simulink model "reaction_pendulum_OBSERVERCOMP"  (R2021b)
settings: Solver=FixedStepDiscrete  StartTime=0.0  StopTime=inf  FixedStep=h  RelTol=1e-3  EnableMultiTasking=on
PreLoadFcn:
  | warning('off','MATLAB:dispatcher:InexactMatch');
InitFcn:
  | hwinit
values from neighbouring files (symbols this model uses):
  A = [0.989609173212  0  0; 0  1  0.01; -0.000301949872013  -0.0950246262215  0.997224421049]    [MATRICES.mat]    (also in SS_11_5.mat = [0.9904  0  0; 0  1  0.01; -9e-05  -0.033262024  0.99812133]; WEAREGOINGHOMEMATRICES.mat = [0.989609173212  0  0; 0  1  0.01; 0.000423899858033  -0.095; current_SS.mat = [0.989609173212  0  0; 0  1  0.01; -9.34612180115e-05  -0.02; dynamicUpdateModel.m = [1.000494318995348 0.010001647563961 2.391143629140888e-07)
  Aeq = [Aeq; Ax0]    [Manual_MPC_Companion.m]    (also in Manual_MPC_Companion_THURSDAY.m = zeros(n * Np, n_total))
  B = [4.20519003073 0 0]    [MATRICES.mat]    (also in SS_11_5.mat = [4.1334 0 0]; current_SS.mat; dynamicUpdateModel.m = [-1.828407620987413e-04; full_dynamics.m = dsys.B)
  beq = zeros(n_total,1)    [Manual_MPC_Companion.m]    (also in Manual_MPC_Companion_THURSDAY.m = zeros(n * Np, 1))
  C = [1 0 0; 0 1 0]    [MeasModel.m]    (also in SS_11_5.mat = [1  0  0; 0  1  0]; current_SS.mat = [1  0  0; 0  1  0]; full_dynamics.m = dsys.C; full_system_ID.m = sys_est.C)
  h = 0.01    [SS_11_5.mat]    (also in hwinit.m)
  H = diag([kron(ones(1,Np), Q) kron(ones(1,Np), R)])    [Manual_MPC_Companion.m]    (also in Manual_MPC_Companion_THURSDAY.m = blkdiag(Qbar, Rbar))
  lb = [-1e6*ones(nx_total,1); -ones(m*Np,1)]    [Manual_MPC_Companion.m]    (also in Manual_MPC_Companion_THURSDAY.m = [-1e6*ones(nx_total, 1); -ones(nu_total, 1)])
  ub = [1e6*ones(nx_total,1); ones(m*Np,1)]    [Manual_MPC_Companion.m]    (also in Manual_MPC_Companion_THURSDAY.m = [ 1e6*ones(nx_total, 1);  ones(nu_total, 1)])
undefined symbols (not defined in the file or in its folder): cThresh, Discrete, E_ref, g_eff, K, k_e, L, magnitude, Time
libraries: sharedTrackingLibrary x1, ctrlSharedLib x1, mpclib x1
settings Model: SimulationMode=external  ExtModeTrigDuration=100000  Creator=user  LastModifiedBy=suray
settings DataIOCC: SaveFormat=Array  SignalLoggingSaveFormat=ModelDataLogs  SaveOutput=off  SignalLogging=off  DSMLogging=off  SaveTime=off  ReturnWorkspaceOutputs=off
settings OptimizationCC: ExpressionDepthLimit=2147483647  LifeSpan=inf
settings DebuggingCC: UnderspecifiedInitializationDetection=Classic  MergeDetectMultiDrivingBlocksExec=none  SolverPrmCheckMsg=warning  FcnCallInpInsideContextMsg=warning  StateNameClashWarn=warning  SFUnexpectedBacktrackingDiag=warning  SFNoUnconditionalDefaultTransitionDiag=warning  SFExecutionAtInitializationDiag=none  ArithmeticOperatorsInVariantConditions=warning
settings HardwareCC: ProdBitPerPointer=32  ProdBitPerSizeT=32  ProdBitPerPtrDiffT=32  ProdLargestAtomicFloat=None  ProdIntDivRoundTo=Undefined  ProdEndianess=Unspecified  ProdWordSize=32  ProdHWDeviceType=32-bit Generic
settings ModelReferenceCC: PropagateSignalLabelsOutOfModel=off
settings SFSimCC: SimUseLocalCustomCode=off  CustomCodeUndefinedFunction=UseInterfaceOnly
settings RTWCC: Description=rpend RTDAC/USB2 (Visual C/C++)  SystemTargetFile=rtcon_rpend_usb2.tlc  TemplateMakefile=rtcon_rpend_vc_usb2_x64.tmf  RTWUseLocalCustomCode=off
settings CodeAppCC: StateflowObjectComments=on
settings STFCustomTargetCC: ModelReferenceCompliant=off  CombineOutputUpdateFcns=on  MatFileLogging=on  GRTInterface=off  SystemTargetFile=rtcon_rpend_usb2.tlc
settings GRTTargetCC: TargetLangStandard=C89/C90 (ANSI)  ModelReferenceCompliant=off  ParMdlRefBuildCompliant=off  CompOptLevelCompliant=off  ConcurrentExecutionCompliant=off  CPPClassGenCompliant=off  UseToolchainInfoCompliant=off  ExtMode=on  ExtModeMexFile=rtcon_ext_comm
settings ConfigComp: CovMetricSettings=dw  CovSaveCumulativeToWorkspaceVar=on  CovSaveSingleToWorkspaceVar=on  CovExternalEMLEnable=off  CovSFcnEnable=off

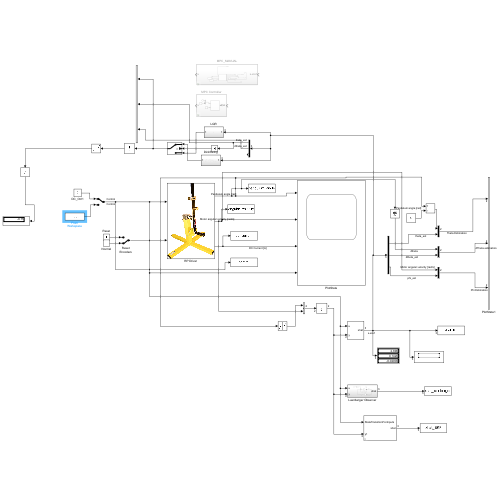
[thumbnail: Simulink's stored preview of the top-level diagram]
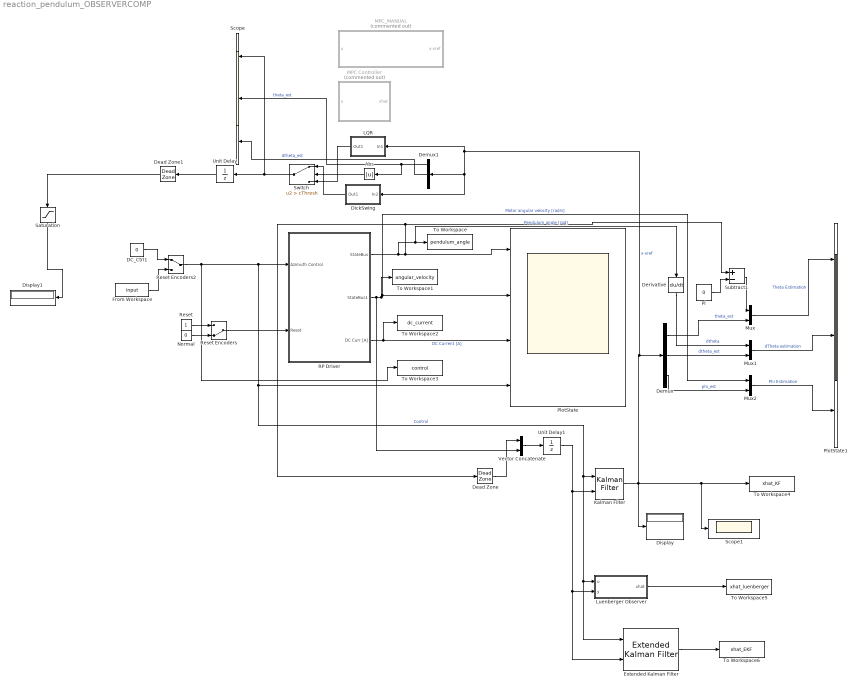
== system reaction_pendulum_OBSERVERCOMP ==
  Abs : Abs
  DC_Ctrl1 : Constant  Value=0
  Dead Zone : DeadZone  LowerValue=0  UpperValue=0.0  SaturateOnIntegerOverflow=on
  Dead Zone1 : DeadZone  LowerValue=0  UpperValue=0  SaturateOnIntegerOverflow=on
  Demux : Demux  Outputs=3
  Demux1 : Demux  Outputs=3
  Derivative : Derivative
  DickSwing : Subsystem
  Display : Display
  Display1 : Display
  Extended Kalman Filter : sharedTrackingLibrary/Extended Kalman Filter  StateTransitionFcn=dynamicUpdateModel  HasStateTransitionJacobianFcn=off  HasAdditiveProcessNoise=Additive  ProcessNoise=diag([0.00001 0.05 0.0001])  HasTimeVaryingProcessNoise=off  HasStateTransitionFcnExtraArgument=1  InitialState=[0;0;0]  InitialStateCovariance=eye(3)  MeasurementFcn1=measModel  HasMeasurementJacobianFcn1=off  HasMeasurementEnablePort1=off  HasAdditiveMeasurementNoise1=Additive  MeasurementNoise1=diag([0.0001 0.01])  HasTimeVaryingMeasurementNoise1=off  HasMeasurementFcnExtraArgument1=0  MeasurementFcn2=myMeasurementFcn  HasMeasurementJacobianFcn2=off  HasMeasurementEnablePort2=off  HasAdditiveMeasurementNoise2=Additive  MeasurementNoise2=1  HasTimeVaryingMeasurementNoise2=off  HasMeasurementFcnExtraArgument2=0  MeasurementFcn3=myMeasurementFcn  HasMeasurementJacobianFcn3=off  HasMeasurementEnablePort3=off  HasAdditiveMeasurementNoise3=Additive  MeasurementNoise3=1  HasTimeVaryingMeasurementNoise3=off  HasMeasurementFcnExtraArgument3=0  MeasurementFcn4=myMeasurementFcn  HasMeasurementJacobianFcn4=off  HasMeasurementEnablePort4=off  HasAdditiveMeasurementNoise4=Additive  MeasurementNoise4=1  HasTimeVaryingMeasurementNoise4=off  HasMeasurementFcnExtraArgument4=0  MeasurementFcn5=myMeasurementFcn  HasMeasurementJacobianFcn5=off  HasMeasurementEnablePort5=off  HasAdditiveMeasurementNoise5=Additive  MeasurementNoise5=1  HasTimeVaryingMeasurementNoise5=off  HasMeasurementFcnExtraArgument5=0  EnableMultirate=off  StateTransitionFcnSampleTime=1  MeasurementFcn1SampleTime=1  MeasurementFcn2SampleTime=1  MeasurementFcn3SampleTime=1  MeasurementFcn4SampleTime=1  MeasurementFcn5SampleTime=1  UseCurrentEstimator=on  OutputStateCovariance=off  DataType=double  SampleTime=h  NumberOfMeasurements=1
      settings: SourceProductBaseCode=AE,PW,CT,DR,TF,ID,LP,NV,AR,RO,RR,UV,VE
  From Workspace : FromWorkspace  VariableName=input
  Kalman Filter : ctrlSharedLib/Kalman Filter  TimeDomain=Discrete-Time  UseCurrentEstimator=on  ModelSource=Individual A, B, C, D matrices  ModelSourceVariable=ss(0.95,1,1,0,1)  A=A  B=B  C=C  D=[0;0]  NumberOfStates=1  NumberOfInputs=1  NumberOfOutputs=1  InitialEstimateSource=Dialog  X0=0  P0=10  UseK=off  UseGH=off  NumberOfProcessNoiseInputs=1  G=1  TimeInvariantG=on  H=0  TimeInvariantH=on  Q=diag([0.00001 0.05 0.0001])  TimeInvariantQ=on  R=diag([0.0001 0.01])  TimeInvariantR=on  N=0  TimeInvariantN=on  AddInputPort=on  AddEnablePort=off  OutputEstimatedY=off  OutputP=off  Ts=-1
  LQR : Subsystem
  Luenberger Observer : Subsystem
  MPC Controller : Subsystem  Commented=on
  MPC_MANUAL : Subsystem  Commented=on
  Mux : Mux  Inputs=2
  Mux1 : Mux  Inputs=2
  Mux2 : Mux  Inputs=2
  Normal : Constant  Value=0
  Pi : Constant  Value=0  OutDataTypeStr=Inherit: Inherit via back propagation
  PlotState : Scope  NumInputPorts=4
  PlotState1 : Scope  NumInputPorts=3
  RP Driver : Subsystem
      mask Display: image(imread('rwp.JPG'))
  Reset : Constant
  Reset Encoders : ManualSwitch  CurrentSetting=0
  Reset Encoders2 : ManualSwitch
  Saturation : Saturate  UpperLimit=1  LowerLimit=-1
  Scope : Scope  NumInputPorts=3
  Scope1 : Scope
  Subtract1 : Sum  Inputs=+-
  Switch : Switch  Criteria=u2 > Threshold  Threshold=cThresh
  To Workspace : ToWorkspace  VariableName=pendulum_angle  SaveFormat=Timeseries  SampleTime=-1
  To Workspace1 : ToWorkspace  VariableName=angular_velocity  SaveFormat=Timeseries  SampleTime=-1
  To Workspace2 : ToWorkspace  VariableName=dc_current  SaveFormat=Timeseries  SampleTime=-1
  To Workspace3 : ToWorkspace  VariableName=control  SaveFormat=Timeseries  SampleTime=-1
  To Workspace4 : ToWorkspace  VariableName=xhat_KF  SaveFormat=Timeseries  SampleTime=-1
  To Workspace5 : ToWorkspace  VariableName=xhat_luenberger  SaveFormat=Timeseries  SampleTime=-1
  To Workspace6 : ToWorkspace  VariableName=xhat_EKF  SaveFormat=Timeseries  SampleTime=-1
  Unit Delay : UnitDelay  SampleTime=0.01
  Unit Delay1 : UnitDelay  SampleTime=0.01
  Vector Concatenate : Concatenate
  wires:
  Normal/1 -> Reset Encoders/2
  Reset/1 -> Reset Encoders/1
  Reset Encoders/1 -> RP Driver/2(Reset)
  RP Driver/3(DC Curr [A]) -> To Workspace2/1, PlotState/3  "DC Current [A]"
  Reset Encoders2/1 -> Kalman Filter/1, Extended Kalman Filter/1, Luenberger Observer/1(u), PlotState/4, RP Driver/1(Azimuth Control), To Workspace3/1  "Control"
  RP Driver/2(StateBus1) -> Vector Concatenate/2, Mux2/1, PlotState/2, To Workspace1/1  "Motor angular velocity [rad/s]"
  RP Driver/1(StateBus) -> Dead Zone/1, Subtract1/1, PlotState/1, Derivative/1, To Workspace/1  "Pendulum angle [rad]"
  Vector Concatenate/1 -> Unit Delay1/1
  Unit Delay1/1 -> Kalman Filter/2, Luenberger Observer/2(y), Extended Kalman Filter/2
  Demux/3 -> Mux2/2  "phi_est"
  Demux/2 -> Mux1/2  "dtheta_est"
  Demux/1 -> Mux/2  "theta_est"
  Derivative/1 -> Mux1/1  "dtheta"
  Mux/1 -> PlotState1/1  "Theta Estimation"
  Mux1/1 -> PlotState1/2  "dTheta estimation"
  Mux2/1 -> PlotState1/3  "Phi Estimation"
  Saturation/1 -> Display1/1
  DC_Ctrl1/1 -> Reset Encoders2/1
  Kalman Filter/1 -> LQR/1(In1), DickSwing/1(In2), Demux1/1, Demux/1, Display/1, Scope1/1, To Workspace4/1  "x-xref"
  Pi/1 -> Subtract1/2
  Subtract1/1 -> Mux/1
  Abs/1 -> Switch/2
  Switch/1 -> Scope/1, Unit Delay/1
  DickSwing/1(Out1) -> Switch/1
  Demux1/1 -> Abs/1, Scope/2  "theta_est"
  Unit Delay/1 -> Dead Zone1/1
  Dead Zone/1 -> Vector Concatenate/1
  Demux1/2 -> Scope/3  "dtheta_est"
  LQR/1(Out1) -> Switch/3
  Dead Zone1/1 -> Saturation/1
  Luenberger Observer/1(xhat) -> To Workspace5/1
  Extended Kalman Filter/1 -> To Workspace6/1
  From Workspace/1 -> Reset Encoders2/2

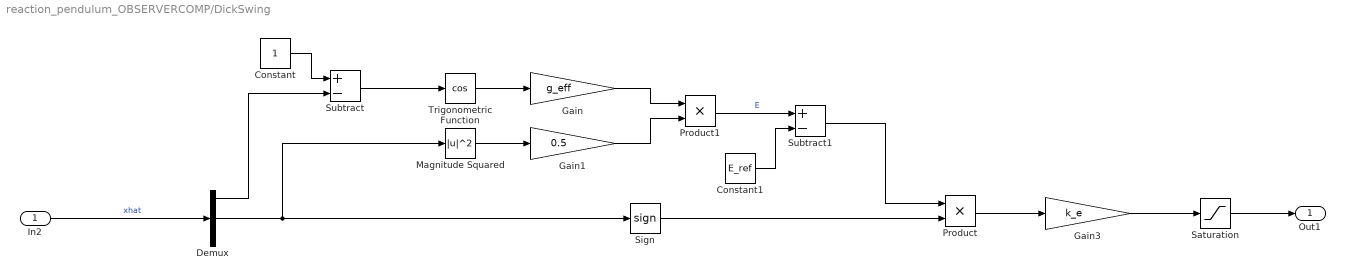
== system reaction_pendulum_OBSERVERCOMP/DickSwing ==
  In2 : Inport
  Constant : Constant
  Constant1 : Constant  Value=E_ref
  Demux : Demux  Outputs=3
  Gain : Gain  Gain=g_eff
  Gain1 : Gain  Gain=0.5
  Gain3 : Gain  Gain=k_e
  Magnitude Squared : Math  Operator=magnitude^2  SaturateOnIntegerOverflow=on
  Product : Product
  Product1 : Product
  Saturation : Saturate  UpperLimit=0.75  LowerLimit=-0.75
  Sign : Signum
  Subtract : Sum  Inputs=+-
  Subtract1 : Sum  Inputs=+-
  Trigonometric Function : Trigonometry  Operator=cos
  Out1 : Outport
  wires:
  In2/1 -> Demux/1  "xhat"
  Trigonometric Function/1 -> Gain/1
  Magnitude Squared/1 -> Gain1/1
  Gain/1 -> Product1/1
  Gain1/1 -> Product1/2
  Constant/1 -> Subtract/1
  Subtract/1 -> Trigonometric Function/1
  Demux/1 -> Subtract/2
  Sign/1 -> Product/2
  Product1/1 -> Subtract1/1  "E"
  Constant1/1 -> Subtract1/2
  Subtract1/1 -> Product/1
  Product/1 -> Gain3/1
  Gain3/1 -> Saturation/1
  Demux/2 -> Magnitude Squared/1, Sign/1
  Saturation/1 -> Out1/1

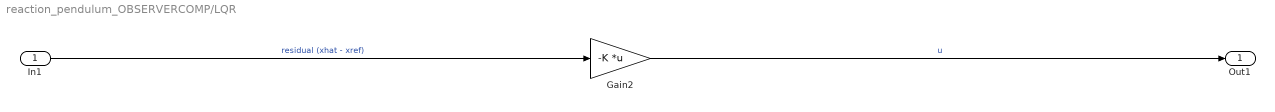
== system reaction_pendulum_OBSERVERCOMP/LQR ==
  In1 : Inport
  Gain2 : Gain  Gain=-K  Multiplication=Matrix(K*u) (u vector)
  Out1 : Outport
  wires:
  In1/1 -> Gain2/1  "residual (xhat - xref)"
  Gain2/1 -> Out1/1  "u"

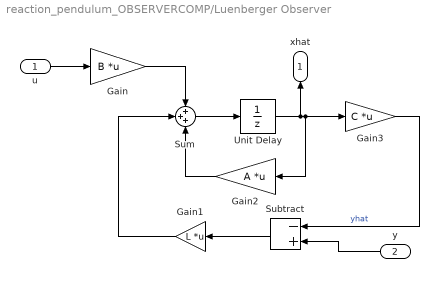
== system reaction_pendulum_OBSERVERCOMP/Luenberger Observer ==
  u : Inport
  y : Inport  Port=2
  Gain : Gain  Gain=B  Multiplication=Matrix(K*u) (u vector)
  Gain1 : Gain  Gain=L  Multiplication=Matrix(K*u) (u vector)
  Gain2 : Gain  Gain=A  Multiplication=Matrix(K*u) (u vector)
  Gain3 : Gain  Gain=C  Multiplication=Matrix(K*u) (u vector)
  Subtract : Sum  Inputs=-+
  Sum : Sum  Inputs=+++
  Unit Delay : UnitDelay  SampleTime=h  HasFrameUpgradeWarning=on
  xhat : Outport
  wires:
  y/1 -> Subtract/2
  Sum/1 -> Unit Delay/1
  Unit Delay/1 -> Gain3/1, Gain2/1, xhat/1
  Gain2/1 -> Sum/3
  u/1 -> Gain/1
  Gain/1 -> Sum/1
  Gain1/1 -> Sum/2
  Gain3/1 -> Subtract/1  "yhat"
  Subtract/1 -> Gain1/1

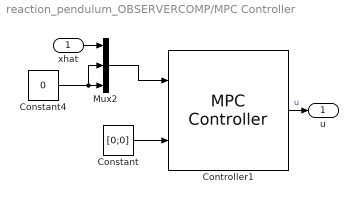
== system reaction_pendulum_OBSERVERCOMP/MPC Controller ==
  xhat : Inport
  Constant : Constant  Value=[0;0]
  Constant4 : Constant  Value=0
  Controller1 : mpclib/MPC Controller  SCDEnableBlockLinearizationSpecification=on  mpcobj=MPC_controller  is_multiple=0  enable_value=0  return_u0=off  updateMPCinCallerWorkspace=on  md_inport=off  mv_inport=off  uref_inport=off  return_cost=off  return_mvseq=off  return_qpstatus=off  return_xseq=off  return_state=off  return_ovseq=off  state_inport=on  umin_inport=off  umax_inport=off  ymin_inport=off  ymax_inport=off  cc_inport=off  ywt_inport=off  uwt_inport=off  duwt_inport=off  rhoeps_inport=off  pm_inport=off  MaximumP=10  HorizonChoice=FixedHorizon  n_ts=0.01  n_p=30  n_mv=1  n_md=0  n_ud=0  n_mo=2  n_uo=0  BlockDataType=double  SampleTimeInherited=off  switch_inport=off
  Mux2 : Mux  Inputs=3
  u : Outport
  wires:
  Controller1/1 -> u/1  "u"
  xhat/1 -> Mux2/1
  Constant4/1 -> Mux2/3, Mux2/2
  Mux2/1 -> Controller1/1
  Constant/1 -> Controller1/2

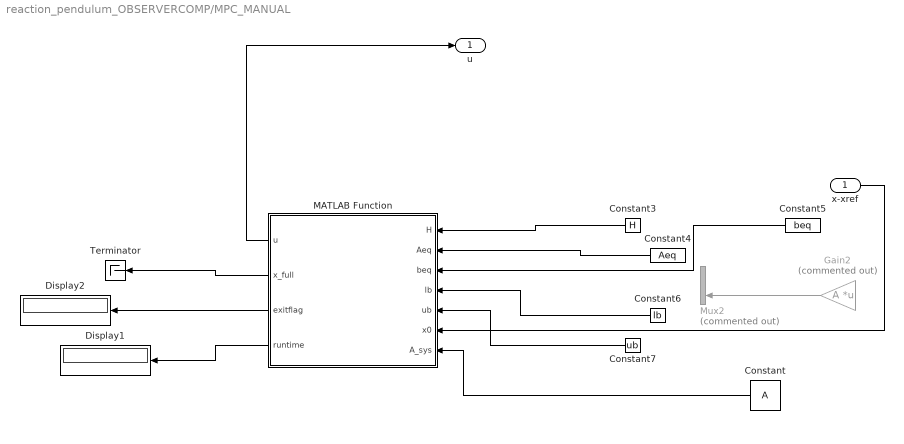
== system reaction_pendulum_OBSERVERCOMP/MPC_MANUAL ==
  x-xref : Inport
  Constant : Constant  Value=A  VectorParams1D=off
  Constant3 : Constant  Value=H
  Constant4 : Constant  Value=Aeq
  Constant5 : Constant  Value=beq
  Constant6 : Constant  Value=lb
  Constant7 : Constant  Value=ub
  Display1 : Display
  Display2 : Display
  Gain2 : Gain  Commented=on  Gain=A  Multiplication=Matrix(K*u) (u vector)
  MATLAB Function : MATLAB Function  TreatAsAtomicUnit=on
  Mux2 : Mux  Commented=on  Inputs=2
  Terminator : Terminator
  u : Outport
  wires:
  Constant3/1 -> MATLAB Function/1(H)
  Constant4/1 -> MATLAB Function/2(Aeq)
  Constant5/1 -> MATLAB Function/3(beq)
  Constant6/1 -> MATLAB Function/4(lb)
  MATLAB Function/3(exitflag) -> Display2/1
  Gain2/1 -> Mux2/2
  Constant7/1 -> MATLAB Function/5(ub)
  MATLAB Function/4(runtime) -> Display1/1
  MATLAB Function/2(x_full) -> Terminator/1
  x-xref/1 -> MATLAB Function/6(x0)
  MATLAB Function/1(u) -> u/1
  Constant/1 -> MATLAB Function/7(A_sys)

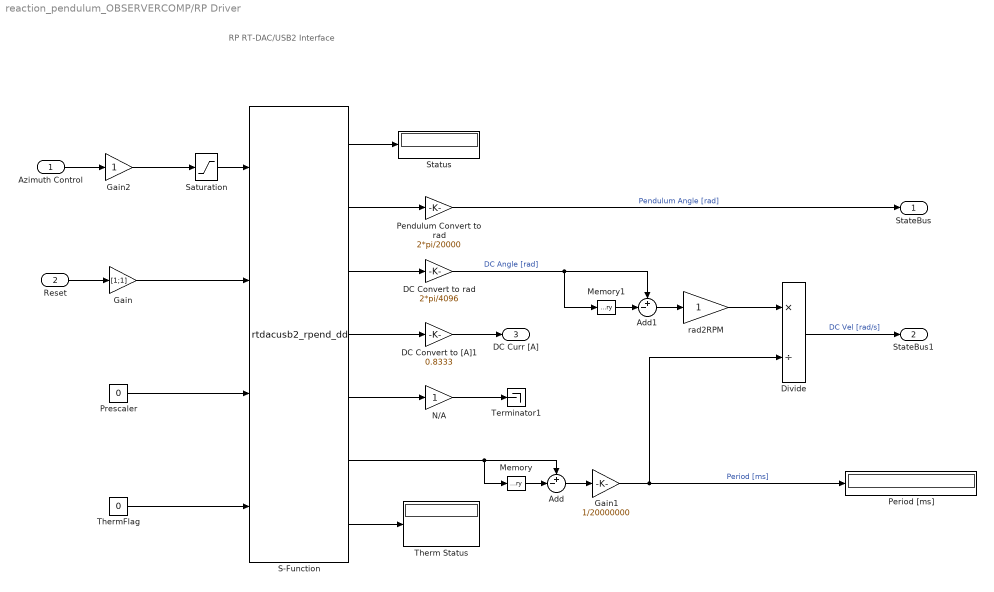
== system reaction_pendulum_OBSERVERCOMP/RP Driver ==
  note: RP RT-DAC/USB2
      | Interface
  Azimuth Control : Inport
  Reset : Inport  Port=2
  Add : Sum  Inputs=+-|
  Add1 : Sum  Inputs=+-|
  DC Convert to [A]1 : Gain  Gain=0.8333  SaturateOnIntegerOverflow=on  OutDataTypeStr=Inherit: Same as input  ParamDataTypeStr=Inherit: Same as input
  DC Convert to rad : Gain  Gain=2*pi/4096  SaturateOnIntegerOverflow=on  OutDataTypeStr=Inherit: Same as input  ParamDataTypeStr=Inherit: Same as input
  Divide : Product  Inputs=*/
  Gain : Gain  Gain=[1;1]
  Gain1 : Gain  Gain=1/20000000
  Gain2 : Gain
  Memory : Memory
  Memory1 : Memory
  N/A : Gain  SaturateOnIntegerOverflow=on  OutDataTypeStr=Inherit: Same as input  ParamDataTypeStr=Inherit: Same as input
  Pendulum Convert to rad : Gain  Gain=2*pi/20000  SaturateOnIntegerOverflow=on  OutDataTypeStr=Inherit: Same as input  ParamDataTypeStr=Inherit: Same as input
  Period [ms] : Display
  Prescaler : Constant  Value=0
  S-Function : S-Function  FunctionName=rtdacusb2_rpend_dd  Parameters=1, h  SFunctionDeploymentMode=off  EnableBusSupport=off
  Saturation : Saturate  UpperLimit=1  LowerLimit=-1
  Status : Display
  Terminator1 : Terminator
  Therm Status : Display
  ThermFlag : Constant  Value=0
  rad2RPM : Gain  SaturateOnIntegerOverflow=on  OutDataTypeStr=Inherit: Same as input  ParamDataTypeStr=Inherit: Same as input
  StateBus : Outport  VectorParamsAs1DForOutWhenUnconnected=off
  StateBus1 : Outport  Port=2  VectorParamsAs1DForOutWhenUnconnected=off
  DC Curr [A] : Outport  Port=3  VectorParamsAs1DForOutWhenUnconnected=off
  wires:
  S-Function/7 -> Therm Status/1
  S-Function/5 -> N/A/1
  S-Function/4 -> DC Convert to [A]1/1
  ThermFlag/1 -> S-Function/4
  Prescaler/1 -> S-Function/3
  Gain/1 -> S-Function/2
  DC Convert to [A]1/1 -> DC Curr [A]/1
  Divide/1 -> StateBus1/1  "DC Vel [rad/s]"
  rad2RPM/1 -> Divide/1
  Add1/1 -> rad2RPM/1
  Memory1/1 -> Add1/2
  N/A/1 -> Terminator1/1
  S-Function/6 -> Add/1, Memory/1
  Gain2/1 -> Saturation/1
  Gain1/1 -> Period [ms]/1, Divide/2  "Period [ms]"
  Add/1 -> Gain1/1
  Memory/1 -> Add/2
  DC Convert to rad/1 -> Add1/1, Memory1/1  "DC Angle [rad]"
  S-Function/3 -> DC Convert to rad/1
  Pendulum Convert to rad/1 -> StateBus/1  "Pendulum Angle [rad]"
  S-Function/2 -> Pendulum Convert to rad/1
  S-Function/1 -> Status/1
  Saturation/1 -> S-Function/1
  Reset/1 -> Gain/1
  Azimuth Control/1 -> Gain2/1

== matlab function reaction_pendulum_OBSERVERCOMP/MPC_MANUAL/MATLAB Function ==
  data: u output size=1; H input; Aeq input; beq input; lb input; ub input; x_full output; exitflag output; runtime output; x0 input; A_sys input
% function [u, x_full, exitflag, runtime] = MPC_short(H, A, b, lb, ub)
% tic
% f  = zeros(size(H,1),1);
% Aineq = zeros(0,size(H,1));
% bineq = zeros(0,1);
% x0 = zeros(size(H,1),1);
% T = size(H,1)/4; % n + m = 4
% 
% opts = optimoptions('quadprog', ...
%     'Algorithm','active-set');
% [x_full, fval, exitflag, output] = quadprog(H, f, Aineq, bineq, A, b, lb, ub, x0, opts);
% u = x_full(3*T+1); % u1
% runtime = toc;

function [u, x_full, exitflag, runtime] = MPC_short(H, Aeq, beq, lb, ub, x0, A_sys)
tic

n = size(A_sys, 1);
T = size(H, 1) / 4;  % Np, since n+m = 4

% Inject current state into the last n rows of beq
beq(end-n+1 : end) = A_sys * x0;

f      = zeros(size(H, 1), 1);
Aineq  = zeros(0, size(H, 1));
bineq  = zeros(0, 1);
x0_qp  = zeros(size(H, 1), 1);

opts = optimoptions('quadprog', 'Algorithm', 'active-set');

[x_full, ~, exitflag, ~] = quadprog(H, f, Aineq, bineq, Aeq, beq, lb, ub, x0_qp, opts);

u = x_full(3*T + 1);  % first control input u_1
runtime = toc;
end
